simulink model "sschdlexBridgeRectifierExample"  (R2023b)
settings: Solver=FixedStepDiscrete  StartTime=0.0  StopTime=0.05  MaxStep=1e-3  RelTol=1e-3  AbsTol=1e-4
InitFcn:
  | Ts=1e-5;
libraries: fl_lib x14, nesl_utility x8, ee_lib x2
CloseFcn:
  | clear Ts;
settings Model: DataTypeOverride=Off  Creator=The MathWorks, Inc.  LastModifiedBy=The MathWorks, Inc.
settings SolverCC: AutoScaleAbsTol=off  AlgebraicLoopSolver=TrustRegion
settings DataIOCC: SaveFormat=Array  SaveOutput=off  SignalLogging=off  DSMLogging=off  SaveTime=off  ReturnWorkspaceOutputs=off
settings OptimizationCC: BlockReduction=off  ConditionallyExecuteInputs=off  DefaultParameterBehavior=Inlined  LifeSpan=inf
settings DebuggingCC: AlgebraicLoopMsg=error  UnderspecifiedInitializationDetection=Classic  MergeDetectMultiDrivingBlocksExec=none  SolverPrmCheckMsg=warning  MultiTaskDSMMsg=warning  MultiTaskCondExecSysMsg=none  SingleTaskRateTransMsg=error  UnconnectedInputMsg=warning  UnconnectedOutputMsg=warning  UnconnectedLineMsg=warning  PregeneratedLibrarySubsystemCodeDiagnostic=none  SFUnexpectedBacktrackingDiag=warning  SFNoUnconditionalDefaultTransitionDiag=warning  SFExecutionAtInitializationDiag=none  ArithmeticOperatorsInVariantConditions=warning
settings HardwareCC: ProdBitPerPointer=32  ProdBitPerSizeT=32  ProdBitPerPtrDiffT=32  ProdLargestAtomicFloat=None  ProdIntDivRoundTo=Undefined  ProdEndianess=Unspecified  ProdWordSize=32  ProdHWDeviceType=ASIC/FPGA->ASIC/FPGA  TargetBitPerPointer=64  TargetBitPerSizeT=64  TargetBitPerPtrDiffT=64  TargetLongLongMode=on  TargetIntDivRoundTo=Zero  TargetEndianess=LittleEndian  TargetWordSize=64  TargetHWDeviceType=Custom Processor->MATLAB Host Computer  ProdEqTarget=off
settings ModelReferenceCC: EnableRefExpFcnMdlSchedulingChecks=on  ModelReferenceNumInstancesAllowed=Single  PropagateSignalLabelsOutOfModel=off
settings SFSimCC: SimUseLocalCustomCode=off  CustomCodeUndefinedFunction=UseInterfaceOnly
settings RTWCC: RTWUseLocalCustomCode=off
settings CodeAppCC: StateflowObjectComments=on
settings GRTTargetCC: TargetLangStandard=C89/C90 (ANSI)
settings ConfigComp: CovMetricSettings=dw  CovSaveCumulativeToWorkspaceVar=on  CovSaveSingleToWorkspaceVar=on  CovExternalEMLEnable=off  CovSFcnEnable=off
settings SimscapeCC: SimscapeNormalizeSystem=off  SimscapeNominalValues="[{\"value\":\"10\",\"unit\":\"V\"},{\"value\":\"1\",\"unit\":\"A\"},{\"value\":\"10\",\"unit\":\"N*m\"},{\"value\":\"10\",\"unit\":\"bar\"},{\"value\":\"100\",\"unit\":\"kJ/kg\"},{\"value\":\"1\",\"unit\":\"kW\"},{\"value\":\"300\",\"unit\":\"K\"},{\"value\":\"100\",\"unit\":\"cm^3/s\"},{\"value\":\"1\",\"unit\":\"kN\"},{\"value\":\"1\",\"unit\":\"g/cm^3\"},{\"value\":\"1\",\"unit\":\"l\"},{\"value\":\"1\",\"unit\":\"cm^2\"},{\"value\":\"60\",\"unit\":\"Hz\"}]"  SimscapeLogSimulationStatistics=on  SimscapeLogLimitData=off

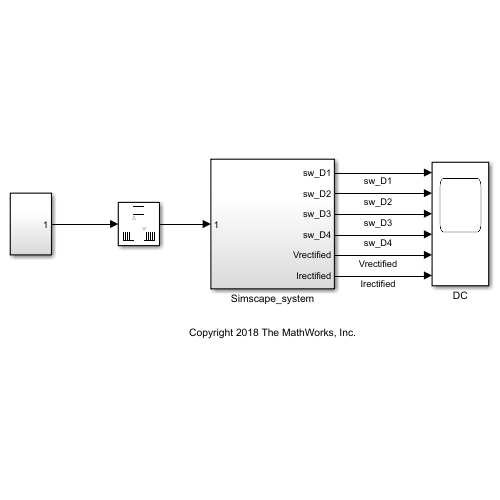
[thumbnail: Simulink's stored preview of the top-level diagram]
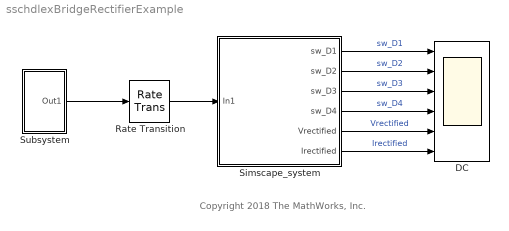
== system sschdlexBridgeRectifierExample ==
  note: Copyright 2018 The MathWorks, Inc.
  DC : Scope  NumInputPorts=6
  Rate Transition : RateTransition
  Simscape_system : Subsystem
  Subsystem : Subsystem
  wires:
  Simscape_system/1(sw_D1) -> DC/1  "sw_D1"
  Simscape_system/2(sw_D2) -> DC/2  "sw_D2"
  Simscape_system/3(sw_D3) -> DC/3  "sw_D3"
  Simscape_system/4(sw_D4) -> DC/4  "sw_D4"
  Simscape_system/5(Vrectified) -> DC/5  "Vrectified"
  Simscape_system/6(Irectified) -> DC/6  "Irectified"
  Rate Transition/1 -> Simscape_system/1(In1)
  Subsystem/1(Out1) -> Rate Transition/1

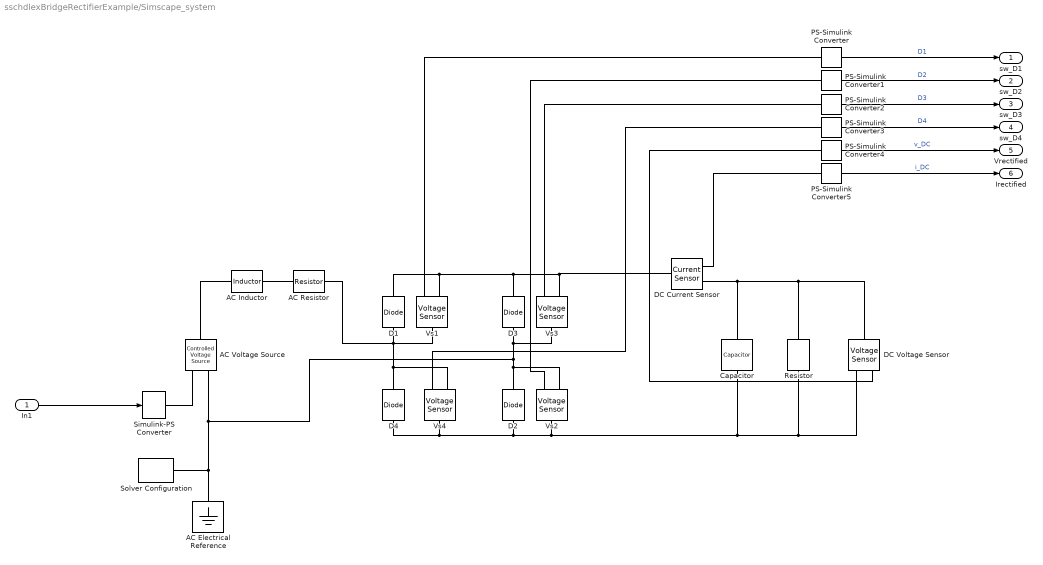
== system sschdlexBridgeRectifierExample/Simscape_system ==
  In1 : Inport
  AC Electrical Reference : fl_lib/Electrical/Electrical Elements/Electrical Reference
  AC Inductor : fl_lib/Electrical/Electrical Elements/Inductor  l=1e-6 H  r=0 Ohm  g=0 1/Ohm  i_specify=off  i_priority=High  i=0 A  i_nominal_specify=off  i_nominal_unit=A  i_nominal_value=1  v_specify=off  v_priority=High  v=0 V  v_nominal_specify=off  v_nominal_unit=V  v_nominal_value=1  i_L_specify=on  i_L_priority=High  i_L=0 A  i_L_nominal_specify=off  i_L_nominal_unit=A  i_L_nominal_value=1
  AC Resistor : fl_lib/Electrical/Electrical Elements/Resistor  R=2 Ohm  i_specify=off  i_priority=High  i=0 A  i_nominal_specify=off  i_nominal_unit=A  i_nominal_value=1  v_specify=off  v_priority=High  v=0 V  v_nominal_specify=off  v_nominal_unit=V  v_nominal_value=1
  AC Voltage Source : fl_lib/Electrical/Electrical Sources/Controlled Voltage Source
  Capacitor : ee_lib/Passive/Capacitor  cap_option=0  c=1e-3 F  Cvec=[1e-05, 1e-06] F  Vvec=[0, 10] V  CV_table_symmetry=1  f_vec=[1, 10] kHz  DFext_vec=[.8, 1.2]  enable_C_tol=0  averaging_period=0 s  C_tol=5  tol_distribution=1  nSigma=4  r=1e-6 Ohm  g=0 1/Ohm  enable_operating_limits=0  enable_faults=ee.enum.enable.no  fault_action=simscape.enum.assert.action.none  Cscale_faulted=100  R_faulted=1e-3 Ohm  G_faulted=0 1/Ohm  tau_fault=1e-3 s  fault_trigger=ee.enum.faults.faultTrigger.temporal  t_fault=1 s  max_permissible_voltage_range=[-100, 100] V  t_fail_on_voltage=1 s  operating_limit_action=2  max_working_voltage_range=[-25, 25] V  power_rating=1 W  i_specify=off  i_priority=None  i=0 A  i_nominal_specify=off  i_nominal_unit=A  i_nominal_value=1  v_specify=off  v_priority=None  v=0 V  v_nominal_specify=off  v_nominal_unit=V  v_nominal_value=1  vc_specify=off  vc_priority=High  vc=0 V  vc_nominal_specify=off  vc_nominal_unit=V  vc_nominal_value=1
  D{1..4} (4 alike) : fl_lib/Electrical/Electrical Elements/Diode  Vf=0.6 V  Ron=0.3 Ohm  Goff=1e-8 1/Ohm  i_specify=off  i_priority=High  i=0 A  i_nominal_specify=off  i_nominal_unit=A  i_nominal_value=1  v_specify=off  v_priority=High  v=0 V  v_nominal_specify=off  v_nominal_unit=V  v_nominal_value=1
  DC Current Sensor : fl_lib/Electrical/Electrical Sensors/Current Sensor
  DC Voltage Sensor : fl_lib/Electrical/Electrical Sensors/Voltage Sensor
  PS-Simulink Converter{,1..5} (6 alike) : nesl_utility/PS-Simulink Converter  PhysicalDomain=network_engine_domain  SubClassName=ps_output  LeftPortType=input  RightPortType=output  PseudoPeriodic=off  Frequencies=[]  VectorFormat=1-D array  Unit=1  AffineConversion=off
  Resistor : ee_lib/Passive/Resistor  R=20 Ohm  enable_R_tol=0  R_tol=5  tol_distribution=1  nSigma=4  enable_operating_limits=0  operating_limit_action=2  power_rating=1 W  max_working_voltage=100 V  enable_faults=ee.enum.enable.no  fault_action=simscape.enum.assert.action.none  R_faulted=inf Ohm  fault_trigger=ee.enum.faults.faultTrigger.temporal  t_fault=1 s  max_permissible_current=1 A  t_fail_on_current=1 s  noise_mode=0  Tdevice=25 degC  sample_time=1e-3 s  repeatability=1  user_seed=0  auto_seed=659950577  power_derating_T1=70 degC  power_derating_T2=155 degC  operating_temperature_range_vec=[-50, 150] degC  alpha=3.93e-3 1/K  Tmeas=25 degC  thermal_mass=100 J/K  temperature_specify=off  temperature_priority=High  temperature=298.15 K  temperature_nominal_specify=off  temperature_nominal_unit=K  temperature_nominal_value=1
  Simulink-PS Converter : nesl_utility/Simulink-PS Converter  PhysicalDomain=network_engine_domain  SubClassName=ps_input  LeftPortType=input  RightPortType=output  PseudoPeriodic=off  Frequencies=[]  NoiseDistribution=none  NoiseParameters=[]  Unit=1  AffineConversion=off  FilteringAndDerivatives=zero  SimscapeFilterOrder=1  InputFilterTimeConstant=0.001  UdotUserProvided=1
  Solver Configuration : nesl_utility/Solver Configuration  PhysicalDomain=network_engine_domain  SubClassName=solver  LeftPortType=input  RightPortType=generic  Tones=[]  Harmonics=[]  SimulateNoise=off  Profile=off  UseLocalSampling=off  EnableSwitchedLinearOptims=off  FrequencyDomain=off  UseCCode=off  RelTol=0.001  AbsTol=1e-06  MinStep=1e-09  ToWorkspace=off  RevertToSquareIcSolve=off  NumHomotopyIterations=100  PhasorMode=off  PhasorModeNumHarmonics=1  ConsistencySolver=NEWTON_FTOL  IndexReductionMethod=DerivativeReplacement  DoDC=off  ResidualTolerance=1e-09  ConsistencyTolSource=GLOBAL  ConsistencyAbsTol=0.001  ConsistencyRelTol=0.001  ConsistencyTolFactor=0.001  UseLocalSolver=on  LocalSolverChoice=NE_BACKWARD_EULER_ADVANCER  ResolveIndetEquations=on  FunctionEvalNumThread=1  LocalSolverSampleTime=Ts  DoFixedCost=on  MaxNonlinIter=3  MaxModeIter=2  ComputeImpulses=off  ImpulseIterations=2  LinearAlgebra=Sparse  LinearAlgebraNumThread=0  EquationFormulation=NE_TIME_EF  DelaysMemoryBudget=1024  AutomaticFiltering=on  FilteringTimeConstant=0.001  PartitionStorageMethod=AS_NEEDED  PartitionMemoryBudget=1024  PartitionMethod=FAST
  Vs{1..4} (4 alike) : fl_lib/Electrical/Electrical Sensors/Voltage Sensor
  sw_D1 : Outport  VectorParamsAs1DForOutWhenUnconnected=off
  sw_D2 : Outport  Port=2  VectorParamsAs1DForOutWhenUnconnected=off
  sw_D3 : Outport  Port=3  VectorParamsAs1DForOutWhenUnconnected=off
  sw_D4 : Outport  Port=4  VectorParamsAs1DForOutWhenUnconnected=off
  Vrectified : Outport  Port=5  VectorParamsAs1DForOutWhenUnconnected=off
  Irectified : Outport  Port=6  VectorParamsAs1DForOutWhenUnconnected=off
  wires:
  PS-Simulink Converter4/1 -> Vrectified/1  "v_DC"
  In1/1 -> Simulink-PS Converter/1
  PS-Simulink Converter3/1 -> sw_D4/1  "D4"
  PS-Simulink Converter1/1 -> sw_D2/1  "D2"
  PS-Simulink Converter/1 -> sw_D1/1  "D1"
  PS-Simulink Converter2/1 -> sw_D3/1  "D3"
  PS-Simulink Converter5/1 -> Irectified/1  "i_DC"
  connections:
  Resistor/RConn1 -- DC Voltage Sensor/RConn2 -- Capacitor/RConn1 -- D4/LConn1 -- Vs4/LConn1 -- D2/LConn1 -- Vs2/LConn1
  AC Electrical Reference/LConn1 -- AC Voltage Source/RConn2 -- Vs3/LConn1 -- D3/LConn1 -- Vs2/RConn2 -- D2/RConn1 -- Solver Configuration/RConn1
  Vs1/LConn1 -- AC Resistor/RConn1 -- Vs4/RConn2 -- D4/RConn1 -- D1/LConn1
  PS-Simulink Converter5/LConn1 -- DC Current Sensor/RConn1
  PS-Simulink Converter4/LConn1 -- DC Voltage Sensor/RConn1
  Simulink-PS Converter/RConn1 -- AC Voltage Source/RConn1
  Vs1/RConn2 -- DC Current Sensor/LConn1 -- Vs3/RConn2 -- D3/RConn1 -- D1/RConn1
  PS-Simulink Converter2/LConn1 -- Vs3/RConn1
  DC Voltage Sensor/LConn1 -- Resistor/LConn1 -- Capacitor/LConn1 -- DC Current Sensor/RConn2
  AC Inductor/RConn1 -- AC Resistor/LConn1
  PS-Simulink Converter3/LConn1 -- Vs4/RConn1
  AC Voltage Source/LConn1 -- AC Inductor/LConn1
  PS-Simulink Converter/LConn1 -- Vs1/RConn1
  PS-Simulink Converter1/LConn1 -- Vs2/RConn1

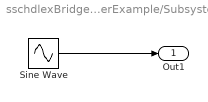
== system sschdlexBridgeRectifierExample/Subsystem ==
  Sine Wave : Sin  Amplitude=100  Frequency=60*2*pi  SampleTime=0
  Out1 : Outport  VectorParamsAs1DForOutWhenUnconnected=off
  wires:
  Sine Wave/1 -> Out1/1
